simulink model "ACC_Demo"  (R2012b)
settings: Solver=ode45  StartTime=0.0  StopTime=150  RelTol=1e-3
undefined symbols (not defined in the file): DiscIntNeverNeededParam, sigbuilder_block
libraries: simulink x3
settings Model: Creator=rima  LastModifiedBy=rima
settings DebuggingCC: LoggingUnavailableSignals=none

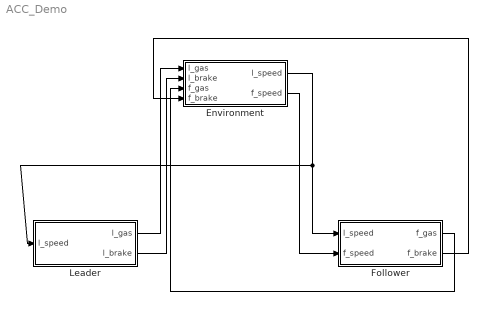
== system ACC_Demo ==
  Environment : Subsystem
  Follower : Subsystem
  Leader : Subsystem
  wires:
  Environment/1(l_speed) -> Follower/1(l_speed), Leader/1(l_speed)
  Environment/2(f_speed) -> Follower/2(f_speed)
  Follower/1(f_gas) -> Environment/3(f_gas)
  Follower/2(f_brake) -> Environment/4(f_brake)
  Leader/1(l_gas) -> Environment/1(l_gas)
  Leader/2(l_brake) -> Environment/2(l_brake)

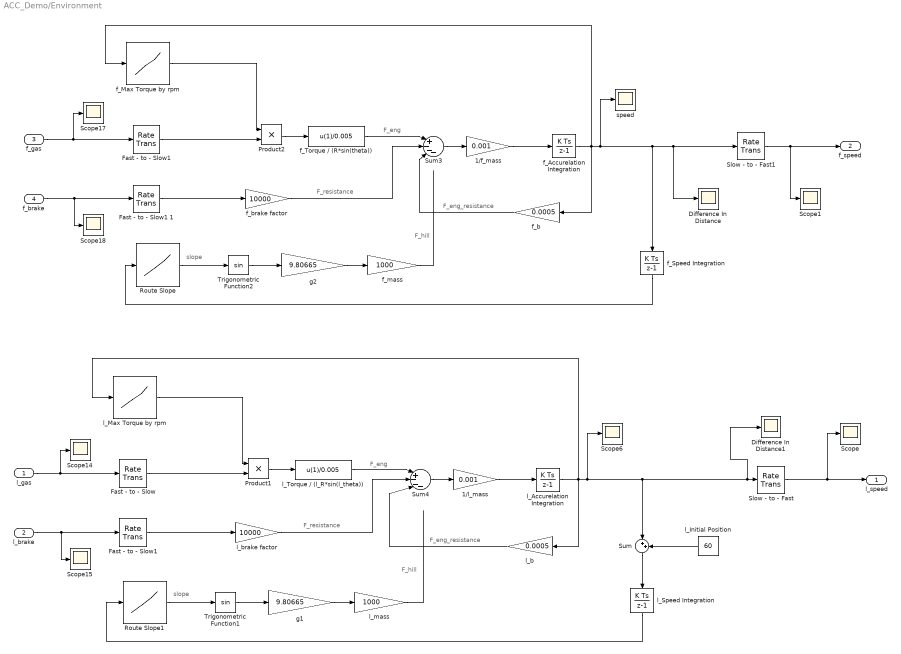
== system ACC_Demo/Environment ==
  note: F_hill
  note: F_eng_resistance
  note: F_resistance
  note: F_eng
  note: F_hill
  note: F_eng_resistance
  note: F_resistance
  note: F_eng
  note: slope
  note: slope
  l_gas : Inport
  l_brake : Inport  Port=2
  f_gas : Inport  Port=3
  f_brake : Inport  Port=4
  1/f_mass : Gain  Gain=0.001
  1/l_mass : Gain  Gain=0.001
  Difference In Distance : Scope
      settings: TimeRange=150  YMin=-150  YMax=150  SaveName=ScopeData5
  Difference In Distance1 : Scope
      settings: TimeRange=150  YMin=-150  YMax=150  SaveName=ScopeData6
  Fast - to - Slow : RateTransition  OutPortSampleTimeMultiple=0.05  OutPortSampleTime=0.1
  Fast - to - Slow1 : RateTransition  OutPortSampleTimeMultiple=0.05  OutPortSampleTime=0.1
  "Fast - to - Slow1 " : RateTransition  OutPortSampleTimeMultiple=0.05  OutPortSampleTime=0.1
  Fast - to - Slow1 1 : RateTransition  OutPortSampleTimeMultiple=0.05  OutPortSampleTime=0.1
  Product1 : Product  RndMeth=Zero
  Product2 : Product  RndMeth=Zero
  Route Slope : Lookup_n-D  NumberOfTableDimensions=1  BreakpointsForDimension1=[0:1000:15000]  Table=[0;pi/3;pi/3;pi/3;pi/5;pi/5;-pi/5;-pi/5;0;pi/4;0;0;0;0;0;0]  RndMeth=Simplest  InputSameDT=on
  Route Slope1 : Lookup_n-D  NumberOfTableDimensions=1  BreakpointsForDimension1=[0:1000:15000]  Table=[0;pi/3;pi/3;pi/3;pi/5;pi/5;-pi/5;-pi/5;0;pi/4;0;0;0;0;0;0]  RndMeth=Simplest  InputSameDT=on
  Scope{,1,6,14..15,17..18} (7 alike) : Scope
      Scope settings: SaveName=ScopeData3
      Scope1 settings: SaveName=ScopeData4
      Scope14 settings: SaveName=ScopeData15
      Scope15 settings: SaveName=ScopeData19
      Scope17 settings: SaveName=ScopeData9
      Scope18 settings: SaveName=ScopeData11
      Scope6 settings: TimeRange=100  YMin=0  YMax=80  SaveName=ScopeData16
  Slow - to - Fast : RateTransition  OutPortSampleTimeMultiple=0.05  OutPortSampleTime=0.05
  Slow - to - Fast1 : RateTransition  OutPortSampleTimeMultiple=0.05  OutPortSampleTime=0.05
  Sum : Sum  Inputs=|++
  Sum3 : Sum  Inputs=|+---
  Sum4 : Sum  Inputs=|+---
  Trigonometric Function1 : Trigonometry
  Trigonometric Function2 : Trigonometry
  f_Accurelation Integration : DiscreteIntegrator  SampleTime=-1  ICPrevOutput=DiscIntNeverNeededParam  ICPrevScaledInput=DiscIntNeverNeededParam
  f_Max Torque by rpm : Lookup_n-D  NumberOfTableDimensions=1  BreakpointsForDimension1=[0;8;20;28;40;60;80;100;120;140;160;180;200]  Table=[165;180;180;170;170;150;115;97;80;70;60;50;40]  RndMeth=Simplest  InputSameDT=on
  f_Speed Integration : DiscreteIntegrator  SampleTime=-1  ICPrevOutput=DiscIntNeverNeededParam  ICPrevScaledInput=DiscIntNeverNeededParam
  f_Torque / (R*sin(theta)) : Fcn  Expr=u(1)/0.005
  f_b : Gain  Gain=0.0005
  f_brake factor : Gain  Gain=10000
  f_mass : Gain  Gain=1000
  g1 : Gain  Gain=9.80665
  g2 : Gain  Gain=9.80665
  l_Accurelation Integration : DiscreteIntegrator  SampleTime=-1  ICPrevOutput=DiscIntNeverNeededParam  ICPrevScaledInput=DiscIntNeverNeededParam
  l_Initial Position : Constant  Value=60
  l_Max Torque by rpm : Lookup_n-D  NumberOfTableDimensions=1  BreakpointsForDimension1=[0;8;20;28;40;60;80;100;120;140;160;180;200]  Table=[165;180;180;170;170;150;115;97;80;70;60;50;40]  RndMeth=Simplest  InputSameDT=on
  l_Speed Integration : DiscreteIntegrator  SampleTime=-1  ICPrevOutput=DiscIntNeverNeededParam  ICPrevScaledInput=DiscIntNeverNeededParam
  l_Torque / (l_R*sin(l_theta)) : Fcn  Expr=u(1)/0.005
  l_b : Gain  Gain=0.0005
  l_brake factor : Gain  Gain=10000
  l_mass : Gain  Gain=1000
  speed : Scope
      settings: TimeRange=100  YMin=0  YMax=80  SaveName=ScopeData36
  l_speed : Outport
  f_speed : Outport  Port=2
  wires:
  l_Initial Position/1 -> Sum/2
  Product1/1 -> l_Torque / (l_R*sin(l_theta))/1
  l_brake factor/1 -> Sum4/2
  Sum4/1 -> 1/l_mass/1
  1/l_mass/1 -> l_Accurelation Integration/1
  l_b/1 -> Sum4/3
  l_gas/1 -> Scope14/1, Fast - to - Slow/1
  l_brake/1 -> Scope15/1, "Fast - to - Slow1 "/1
  l_Torque / (l_R*sin(l_theta))/1 -> Sum4/1
  Fast - to - Slow/1 -> Product1/2
  "Fast - to - Slow1 "/1 -> l_brake factor/1
  l_Accurelation Integration/1 -> l_Max Torque by rpm/1, l_b/1, Difference In Distance1/1, Slow - to - Fast/1, Sum/1, Scope6/1
  Slow - to - Fast/1 -> Scope/1, l_speed/1
  l_Max Torque by rpm/1 -> Product1/1
  Product2/1 -> f_Torque / (R*sin(theta))/1
  f_brake factor/1 -> Sum3/2
  Sum3/1 -> 1/f_mass/1
  1/f_mass/1 -> f_Accurelation Integration/1
  f_b/1 -> Sum3/3
  f_gas/1 -> Scope17/1, Fast - to - Slow1/1
  f_brake/1 -> Scope18/1, Fast - to - Slow1 1/1
  f_Accurelation Integration/1 -> f_Max Torque by rpm/1, f_b/1, f_Speed Integration/1, Difference In Distance/1, Slow - to - Fast1/1, speed/1
  f_Speed Integration/1 -> Route Slope/1
  Route Slope/1 -> Trigonometric Function2/1
  g2/1 -> f_mass/1
  Trigonometric Function2/1 -> g2/1
  f_mass/1 -> ?
  f_Torque / (R*sin(theta))/1 -> Sum3/1
  Fast - to - Slow1/1 -> Product2/2
  Fast - to - Slow1 1/1 -> f_brake factor/1
  Slow - to - Fast1/1 -> Scope1/1, f_speed/1
  f_Max Torque by rpm/1 -> Product2/1
  l_Speed Integration/1 -> Route Slope1/1
  Route Slope1/1 -> Trigonometric Function1/1
  g1/1 -> l_mass/1
  Trigonometric Function1/1 -> g1/1
  l_mass/1 -> ?
  Sum/1 -> l_Speed Integration/1

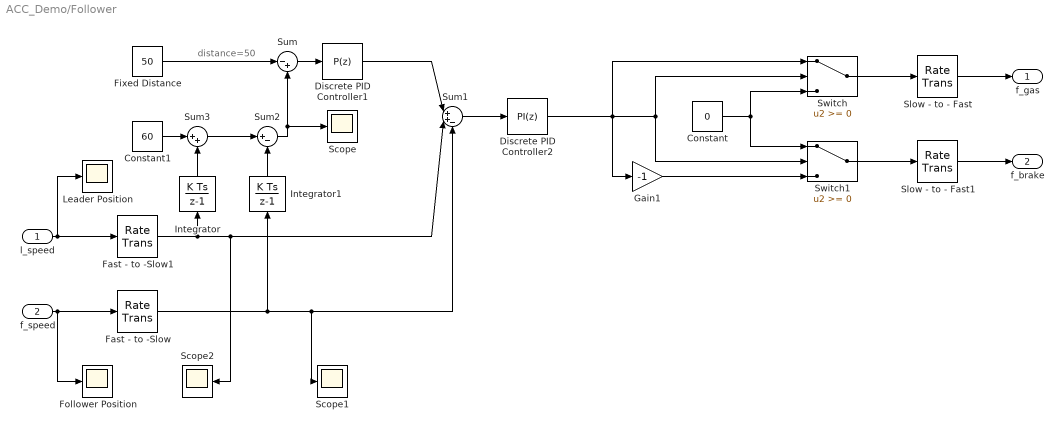
== system ACC_Demo/Follower ==
  note: distance=50
  l_speed : Inport
  f_speed : Inport  Port=2
  Constant : Constant  Value=0
  Constant1 : Constant  Value=60
  Discrete PID Controller1 : simulink/Continuous/PID Controller  Controller=P  TimeDomain=Discrete-time  SampleTime=-1  IntegratorMethod=Forward Euler  FilterMethod=Forward Euler  Form=Parallel  P=0.193  I=0.2  D=0.0001  N=100  InitialConditionSource=internal  InitialConditionForIntegrator=0  InitialConditionForFilter=0  ExternalReset=none  LimitOutput=off  UpperSaturationLimit=1  LowerSaturationLimit=-1  LinearizeAsGain=off  AntiWindupMode=none  Kb=1  TrackingMode=off  Kt=1  PParamMin=[]  PParamMax=[]  IParamMin=[]  IParamMax=[]  DParamMin=[]  DParamMax=[]  NParamMin=[]  NParamMax=[]  KbParamMin=[]  KbParamMax=[]  KtParamMin=[]  KtParamMax=[]  POutMin=[]  POutMax=[]  IOutMin=[]  IOutMax=[]  DOutMin=[]  DOutMax=[]  NOutMin=[]  NOutMax=[]  KbOutMin=[]  KbOutMax=[]  KtOutMin=[]  KtOutMax=[]  IntegratorOutMin=[]  IntegratorOutMax=[]  FilterOutMin=[]  FilterOutMax=[]  SumOutMin=[]  SumOutMax=[]  SumI1OutMin=[]  SumI1OutMax=[]  SumI2OutMin=[]  SumI2OutMax=[]  SumI3OutMin=[]  SumI3OutMax=[]  SumDOutMin=[]  SumDOutMax=[]  SaturationOutMin=[]  SaturationOutMax=[]  IntegratorContinuousStateAttributes=''  IntegratorStateMustResolveToSignalObject=off  IntegratorRTWStateStorageClass=Auto  FilterContinuousStateAttributes=''  FilterStateMustResolveToSignalObject=off  FilterRTWStateStorageClass=Auto
  Discrete PID Controller2 : simulink/Continuous/PID Controller  Controller=PI  TimeDomain=Discrete-time  SampleTime=-1  IntegratorMethod=Forward Euler  FilterMethod=Forward Euler  Form=Parallel  P=0.12631  I=0.001  D=0  N=100  InitialConditionSource=internal  InitialConditionForIntegrator=0  InitialConditionForFilter=0  ExternalReset=none  LimitOutput=on  UpperSaturationLimit=1  LowerSaturationLimit=-1  LinearizeAsGain=off  AntiWindupMode=back-calculation  Kb=0.01  TrackingMode=off  Kt=1  PParamMin=[]  PParamMax=[]  IParamMin=[]  IParamMax=[]  DParamMin=[]  DParamMax=[]  NParamMin=[]  NParamMax=[]  KbParamMin=[]  KbParamMax=[]  KtParamMin=[]  KtParamMax=[]  POutMin=[]  POutMax=[]  IOutMin=[]  IOutMax=[]  DOutMin=[]  DOutMax=[]  NOutMin=[]  NOutMax=[]  KbOutMin=[]  KbOutMax=[]  KtOutMin=[]  KtOutMax=[]  IntegratorOutMin=[]  IntegratorOutMax=[]  FilterOutMin=[]  FilterOutMax=[]  SumOutMin=[]  SumOutMax=[]  SumI1OutMin=[]  SumI1OutMax=[]  SumI2OutMin=[]  SumI2OutMax=[]  SumI3OutMin=[]  SumI3OutMax=[]  SumDOutMin=[]  SumDOutMax=[]  SaturationOutMin=[]  SaturationOutMax=[]  IntegratorContinuousStateAttributes=''  IntegratorStateMustResolveToSignalObject=off  IntegratorRTWStateStorageClass=Auto  FilterContinuousStateAttributes=''  FilterStateMustResolveToSignalObject=off  FilterRTWStateStorageClass=Auto
  Fast - to -Slow : RateTransition  OutPortSampleTimeMultiple=0.05  OutPortSampleTime=0.1
  Fast - to -Slow1 : RateTransition  OutPortSampleTimeMultiple=0.05  OutPortSampleTime=0.1
  Fixed Distance : Constant  Value=50
  Follower Position : Scope
      settings: SaveName=ScopeData44
  Gain1 : Gain  Gain=-1
  Integrator : DiscreteIntegrator  SampleTime=-1  ICPrevOutput=DiscIntNeverNeededParam  ICPrevScaledInput=DiscIntNeverNeededParam
  Integrator1 : DiscreteIntegrator  SampleTime=-1  ICPrevOutput=DiscIntNeverNeededParam  ICPrevScaledInput=DiscIntNeverNeededParam
  Leader Position : Scope
      settings: SaveName=ScopeData14
  Scope : Scope
  Scope1 : Scope
  Scope2 : Scope
      settings: SaveName=ScopeData2
  Slow - to - Fast : RateTransition  OutPortSampleTimeMultiple=0.05  OutPortSampleTime=0.05
  Slow - to - Fast1 : RateTransition  OutPortSampleTimeMultiple=0.05  OutPortSampleTime=0.05
  Sum : Sum  Inputs=|-+
  Sum1 : Sum  Inputs=|++-
  Sum2 : Sum  Inputs=|+-
  Sum3 : Sum  Inputs=|++
  Switch : Switch
  Switch1 : Switch
  f_gas : Outport
  f_brake : Outport  Port=2
  wires:
  Fixed Distance/1 -> Sum/1
  f_speed/1 -> Fast - to -Slow/1, Follower Position/1
  l_speed/1 -> Fast - to -Slow1/1, Leader Position/1
  Sum/1 -> Discrete PID Controller1/1
  Discrete PID Controller2/1 -> Gain1/1, Switch/2, Switch1/2, Switch/1
  Gain1/1 -> Switch1/3
  Switch/1 -> Slow - to - Fast/1
  Constant/1 -> Switch/3, Switch1/1
  Switch1/1 -> Slow - to - Fast1/1
  Slow - to - Fast/1 -> f_gas/1
  Slow - to - Fast1/1 -> f_brake/1
  Sum2/1 -> Sum/2, Scope/1
  Discrete PID Controller1/1 -> Sum1/1
  Fast - to -Slow/1 -> Integrator1/1, Scope1/1, Sum1/3
  Sum1/1 -> Discrete PID Controller2/1
  Fast - to -Slow1/1 -> Scope2/1, Sum1/2, Integrator/1
  Integrator1/1 -> Sum2/2
  Integrator/1 -> Sum3/2
  Constant1/1 -> Sum3/1
  Sum3/1 -> Sum2/1

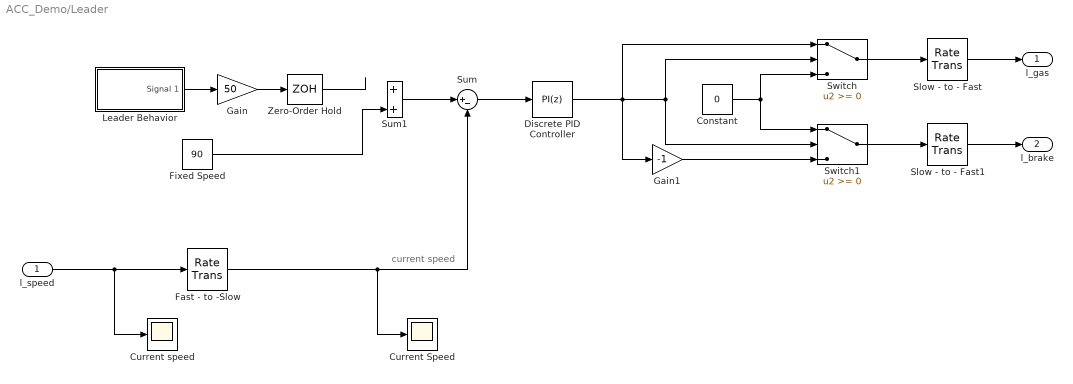
== system ACC_Demo/Leader ==
  note: current speed
  l_speed : Inport
  Constant : Constant  Value=0
  Current Speed : Scope
      settings: TimeRange=10  SaveName=ScopeData25
  Current speed : Scope
      settings: SaveName=ScopeData31
  Discrete PID Controller : simulink/Continuous/PID Controller  Controller=PI  TimeDomain=Discrete-time  SampleTime=-1  IntegratorMethod=Forward Euler  FilterMethod=Forward Euler  Form=Parallel  P=0.05  I=0.000228325  D=0  N=100  InitialConditionSource=internal  InitialConditionForIntegrator=0  InitialConditionForFilter=0  ExternalReset=none  LimitOutput=on  UpperSaturationLimit=1  LowerSaturationLimit=-1  LinearizeAsGain=off  AntiWindupMode=back-calculation  Kb=0.01  TrackingMode=off  Kt=1  PParamMin=[]  PParamMax=[]  IParamMin=[]  IParamMax=[]  DParamMin=[]  DParamMax=[]  NParamMin=[]  NParamMax=[]  KbParamMin=[]  KbParamMax=[]  KtParamMin=[]  KtParamMax=[]  POutMin=[]  POutMax=[]  IOutMin=[]  IOutMax=[]  DOutMin=[]  DOutMax=[]  NOutMin=[]  NOutMax=[]  KbOutMin=[]  KbOutMax=[]  KtOutMin=[]  KtOutMax=[]  IntegratorOutMin=[]  IntegratorOutMax=[]  FilterOutMin=[]  FilterOutMax=[]  SumOutMin=[]  SumOutMax=[]  SumI1OutMin=[]  SumI1OutMax=[]  SumI2OutMin=[]  SumI2OutMax=[]  SumI3OutMin=[]  SumI3OutMax=[]  SumDOutMin=[]  SumDOutMax=[]  SaturationOutMin=[]  SaturationOutMax=[]  IntegratorContinuousStateAttributes=''  IntegratorStateMustResolveToSignalObject=off  IntegratorRTWStateStorageClass=Auto  FilterContinuousStateAttributes=''  FilterStateMustResolveToSignalObject=off  FilterRTWStateStorageClass=Auto
  Fast - to -Slow : RateTransition  OutPortSampleTimeMultiple=0.05  OutPortSampleTime=0.1
  Fixed Speed : Constant  Value=90  SampleTime=-1
  Gain : Gain  Gain=50
  Gain1 : Gain  Gain=-1
  Leader Behavior : Subsystem  Tag=STV Subsys  LoadFcn=sigbuilder_block('load');  StartFcn=sigbuilder_block('start');  StopFcn=sigbuilder_block('stop');  ClipboardFcn=sigbuilder_block('clipboard');  mask(Sigbuilder block){}
      mask help: Simulink:masks:SigbuilderBlock_MD
      mask init:
      | if ~strcmp(get_param(bdroot(gcbh),'SimulationStatus'),'stopped') tuvar = sigbuilder_block('maskInit'); end
      settings: CopyFcn=sigbuilder_block('copy');  DeleteFcn=sigbuilder_block('delete');  ModelCloseFcn=sigbuilder_block('modelClose');  PreSaveFcn=sigbuilder_block('preSave');  PauseFcn=sigbuilder_block('pause');  ContinueFcn=sigbuilder_block('continue');  NameChangeFcn=sigbuilder_block('namechange');  OpenFcn=sigbuilder_block('open',[224.25 370.5 550.5 399.75 ]);  CloseFcn=sigbuilder_block('close');
      mask Display: plot(0, 0, 100, 100,[2, 2, 32, 32, 2], [68, 8, 8, 68, 68],[32, 2], [38, 38], [32, 19, 2],[53, 60, 44], [32, 17, 17, 2],[16, 16, 31, 31]);txt = getActiveGroup(gcbh);text(2, 100, txt,'verticalAlignment', 'top');
  Slow - to - Fast : RateTransition  OutPortSampleTimeMultiple=0.05  OutPortSampleTime=0.05
  Slow - to - Fast1 : RateTransition  OutPortSampleTimeMultiple=0.05  OutPortSampleTime=0.05
  Sum : Sum  Inputs=|+-
  Sum1 : Sum  Inputs=|++
  Switch : Switch
  Switch1 : Switch
  Zero-Order Hold : ZeroOrderHold  SampleTime=0.2
  l_gas : Outport
  l_brake : Outport  Port=2
  wires:
  Fast - to -Slow/1 -> Current Speed/1, Sum/2
  Discrete PID Controller/1 -> Switch/1, Switch/2, Switch1/2, Gain1/1
  Gain1/1 -> Switch1/3
  Switch/1 -> Slow - to - Fast/1
  Constant/1 -> Switch/3, Switch1/1
  Switch1/1 -> Slow - to - Fast1/1
  l_speed/1 -> Fast - to -Slow/1, Current speed/1
  Sum/1 -> Discrete PID Controller/1
  Slow - to - Fast/1 -> l_gas/1
  Slow - to - Fast1/1 -> l_brake/1
  Leader Behavior/1(Signal 1) -> Gain/1
  Gain/1 -> Zero-Order Hold/1
  Fixed Speed/1 -> Sum1/2
  Sum1/1 -> Sum/1
  Zero-Order Hold/1 -> ?

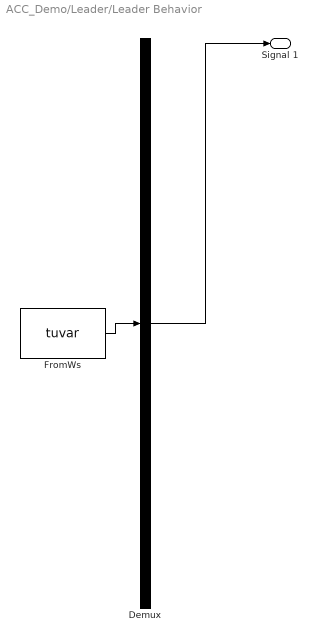
== system ACC_Demo/Leader/Leader Behavior ==
  Demux : Demux  Tag=STV Demux  Outputs=1
  FromWs : FromWorkspace  Tag=STV FromWs  VariableName=tuvar  SampleTime=0
      SigBuilderData=|
      | common.afterFinalStr = 'Extrapolate'
      | common.sampleTime = 0
      | dataSet.timeRange = [0 150]
      | dataSet.name = 'Group 1'
      | sbobj.Groups.Name = 'Group 1'
      | sbobj.Groups.Signals.Name = 'Signal 1'
      | sbobj.Groups.Signals.XData = [0 30 50 50 70 150]
      | sbobj.Groups.Signals.YData = [0 0 1.01 -1.01 0 0]
      | sbobj.Groups.TimeRange = [0 150]
  Signal 1 : Outport  Tag=STV Outport
  wires:
  Demux/1 -> Signal 1/1
  FromWs/1 -> Demux/1
